simulink model "A_Working_project"  (R2025a)
settings: Solver=ode45  StartTime=0.0  StopTime=10  RelTol=1e-3
model workspace (MAT data in the model file):
  Sig = Simulink.Signal
  Sig.Dimensions = -1
  Sig.DimensionsMode = 'auto'
  Sig.Complexity = 'auto'
  Sig.SampleTime = -1
  Sig.SamplingMode = 'auto'
  Sig.DataType = 'auto'
  T = 0.1
  g = 9.8
values from neighbouring files (symbols this model uses):
  kd = 1.187    [final_coffs.mat]
  ki = 0.001    [final_coffs.mat]
  kp = 1.397    [final_coffs.mat]
  Lx = 0.07    [final_coffs.mat]
  Ly = 0.07    [final_coffs.mat]
  rM = 0.03    [final_coffs.mat]
libraries: simulink_extras x2
settings Model: Creator=eid16  LastModifiedBy=eid16

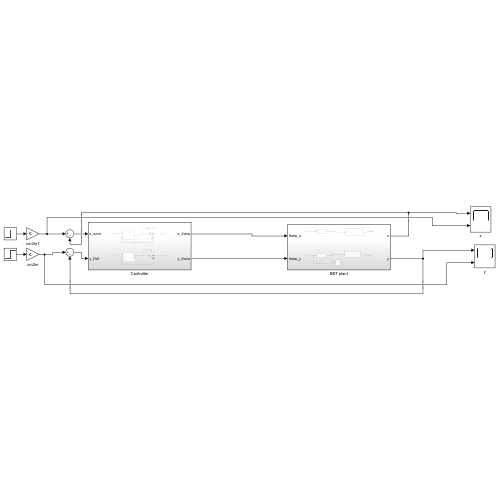
[thumbnail: Simulink's stored preview of the top-level diagram]
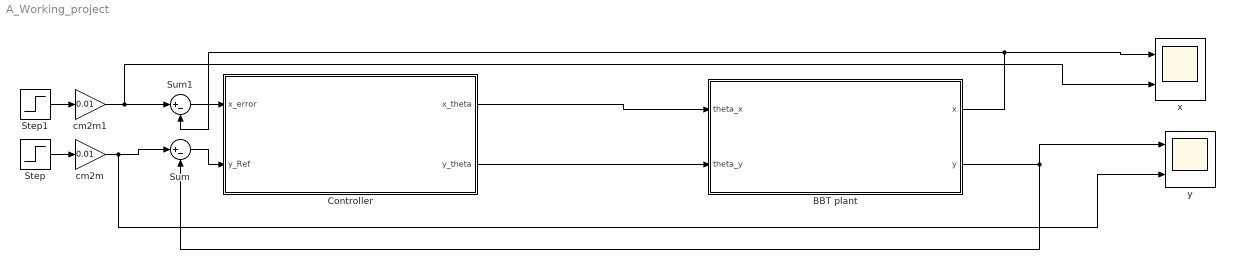
== system A_Working_project ==
  BBT plant : Subsystem
  Controller : Subsystem
  Step : Step  Time=0  After=8  SampleTime=0  ZeroCross=off
  Step1 : Step  Time=0  After=8  SampleTime=0  ZeroCross=off
  Sum : Sum  Inputs=|+-
  Sum1 : Sum  Inputs=|+-
  cm2m : Gain  Gain=0.01
  cm2m1 : Gain  Gain=0.01
  x : Scope  NumInputPorts=2
      settings: ActiveDisplayYMinimum=-0.010000828613582549  ActiveDisplayYMaximum=0.085704430373965509  DataLoggingVariableName=ScopeData2
  y : Scope  NumInputPorts=2
      settings: ActiveDisplayYMinimum=-0.010000509256546551  ActiveDisplayYMaximum=0.090004583308918973
  wires:
  BBT plant/1(x) -> x/1, Sum1/2
  Step/1 -> cm2m/1
  Sum/1 -> Controller/2(y_Ref)
  BBT plant/2(y) -> y/1, Sum/2
  Controller/2(y_theta) -> BBT plant/2(theta_y)
  Step1/1 -> cm2m1/1
  Sum1/1 -> Controller/1(x_error)
  cm2m/1 -> y/2, Sum/1
  cm2m1/1 -> x/2, Sum1/1
  Controller/1(x_theta) -> BBT plant/1(theta_x)

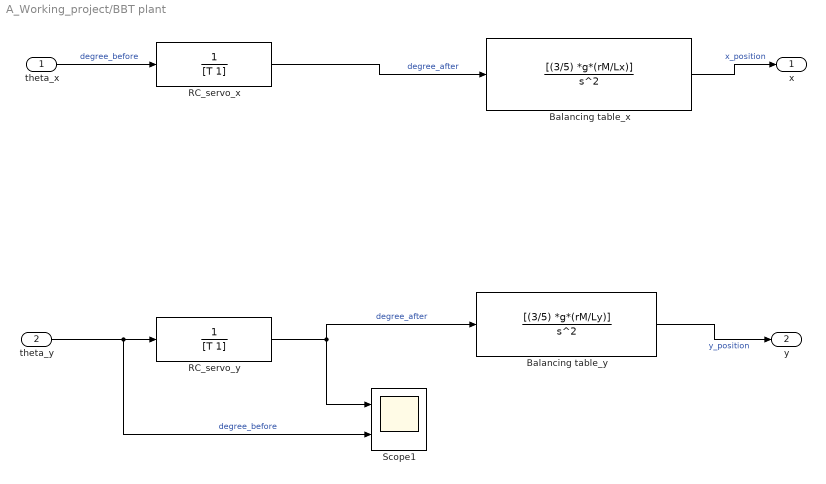
== system A_Working_project/BBT plant ==
  theta_x : Inport
  theta_y : Inport  Port=2
  Balancing table_x : TransferFcn  Numerator=[(3/5) *g*(rM/Lx)]  Denominator=[1 0 0 ]
  Balancing table_y : TransferFcn  Numerator=[(3/5) *g*(rM/Ly)]  Denominator=[1 0 0 ]
  RC_servo_x : TransferFcn  Denominator=[T 1]
  RC_servo_y : TransferFcn  Denominator=[T 1]
  Scope1 : Scope  NumInputPorts=2
  x : Outport
  y : Outport  Port=2
  wires:
  theta_x/1 -> RC_servo_x/1  "degree_before"
  theta_y/1 -> Scope1/2, RC_servo_y/1  "degree_before"
  RC_servo_x/1 -> Balancing table_x/1  "degree_after"
  RC_servo_y/1 -> Balancing table_y/1, Scope1/1  "degree_after"
  Balancing table_y/1 -> y/1  "y_position"
  Balancing table_x/1 -> x/1  "x_position"

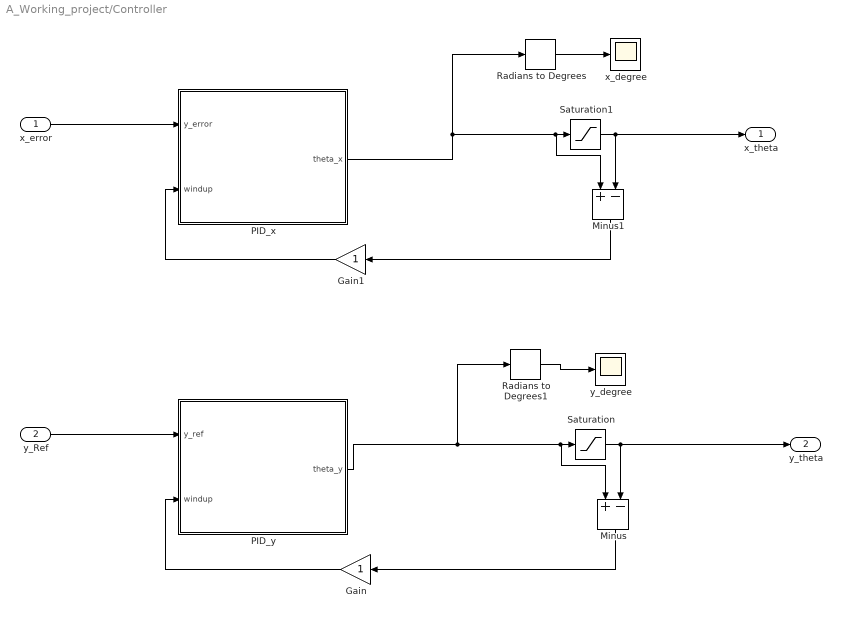
== system A_Working_project/Controller ==
  x_error : Inport
  y_Ref : Inport  Port=2
  Gain : Gain
  Gain1 : Gain
  Minus : Sum  Inputs=+-
  Minus1 : Sum  Inputs=+-
  PID_x : Subsystem
  PID_y : Subsystem
  Radians to Degrees : simulink_extras/Transformations/Radians to Degrees
  Radians to Degrees1 : simulink_extras/Transformations/Radians to Degrees
  Saturation : Saturate  UpperLimit=1  LowerLimit=-1
  Saturation1 : Saturate  UpperLimit=1  LowerLimit=-1
  x_degree : Scope
      settings: ActiveDisplayYMinimum=-0.73658266905448522  ActiveDisplayYMaximum=2.2151758521171652  DataLoggingVariableName=ScopeData3
  y_degree : Scope
      settings: ActiveDisplayYMinimum=-27.898226301117479  ActiveDisplayYMaximum=84.5871337853968  DataLoggingVariableName=ScopeData5
  x_theta : Outport
  y_theta : Outport  Port=2
  wires:
  y_Ref/1 -> PID_y/1(y_ref)
  Gain/1 -> PID_y/2(windup)
  Minus/1 -> Gain/1
  Saturation/1 -> y_theta/1, Minus/2
  PID_y/1(theta_y) -> Radians to Degrees1/1, Minus/1, Saturation/1
  Gain1/1 -> PID_x/2(windup)
  x_error/1 -> PID_x/1(y_error)
  Minus1/1 -> Gain1/1
  PID_x/1(theta_x) -> Radians to Degrees/1, Minus1/1, Saturation1/1
  Saturation1/1 -> x_theta/1, Minus1/2
  Radians to Degrees/1 -> x_degree/1
  Radians to Degrees1/1 -> y_degree/1

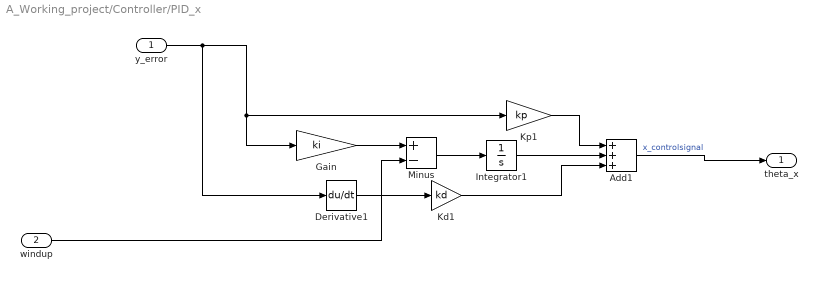
== system A_Working_project/Controller/PID_x ==
  y_error : Inport
  windup : Inport  Port=2
  Add1 : Sum  Inputs=+++
  Derivative1 : Derivative
  Gain : Gain  Gain=ki
  Integrator1 : Integrator
  Kd1 : Gain  Gain=kd
  Kp1 : Gain  Gain=kp
  Minus : Sum  Inputs=+-
  theta_x : Outport
  wires:
  Integrator1/1 -> Add1/2
  Kd1/1 -> Add1/3
  Add1/1 -> theta_x/1  "x_controlsignal"
  Kp1/1 -> Add1/1
  Gain/1 -> Minus/1
  Minus/1 -> Integrator1/1
  windup/1 -> Minus/2
  Derivative1/1 -> Kd1/1
  y_error/1 -> Derivative1/1, Gain/1, Kp1/1

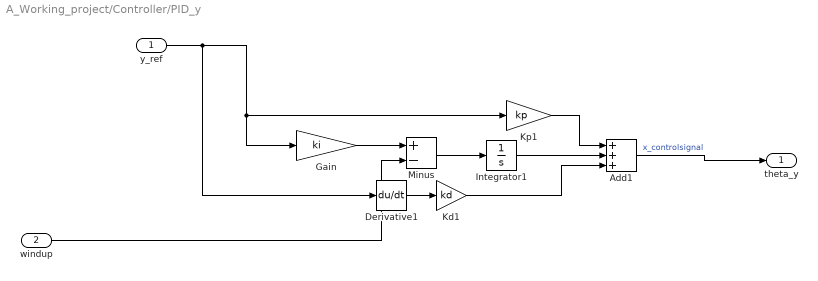
== system A_Working_project/Controller/PID_y ==
  y_ref : Inport
  windup : Inport  Port=2
  Add1 : Sum  Inputs=+++
  Derivative1 : Derivative
  Gain : Gain  Gain=ki
  Integrator1 : Integrator
  Kd1 : Gain  Gain=kd
  Kp1 : Gain  Gain=kp
  Minus : Sum  Inputs=+-
  theta_y : Outport
  wires:
  Integrator1/1 -> Add1/2
  Kd1/1 -> Add1/3
  Add1/1 -> theta_y/1  "x_controlsignal"
  Kp1/1 -> Add1/1
  Gain/1 -> Minus/1
  Minus/1 -> Integrator1/1
  windup/1 -> Minus/2
  y_ref/1 -> Derivative1/1, Gain/1, Kp1/1
  Derivative1/1 -> Kd1/1
